simulink model "DC_MOTOR"  (R2016a)
settings: Solver=VariableStepAuto  StartTime=0.0  StopTime=tend  RelTol=1e-3
values from neighbouring files (symbols this model uses):
  c_M = 1.0    (= 1)    [DCTEST.m]    (also in a71test.m)
  J_A = 2.0    (= 2)    [DCTEST.m]    (also in a71test.m)
  L_A = 0.15    [DCTEST.m]    (also in a71test.m)
  Phi = 1.5    [DCTEST.m]    (also in a71test.m)
  R_A = 2.0    (= 2)    [DCTEST.m]    (also in a71test.m)
  t_ML_step = 12    [DCTEST.m]    (also in a71test.m = 3)
  t_u_A_step = 2    [DCTEST.m]
  u_A = 20    [DCTEST.m]    (also in a71test.m)
settings Model: Creator=mam1205  LastModifiedBy=mam1205

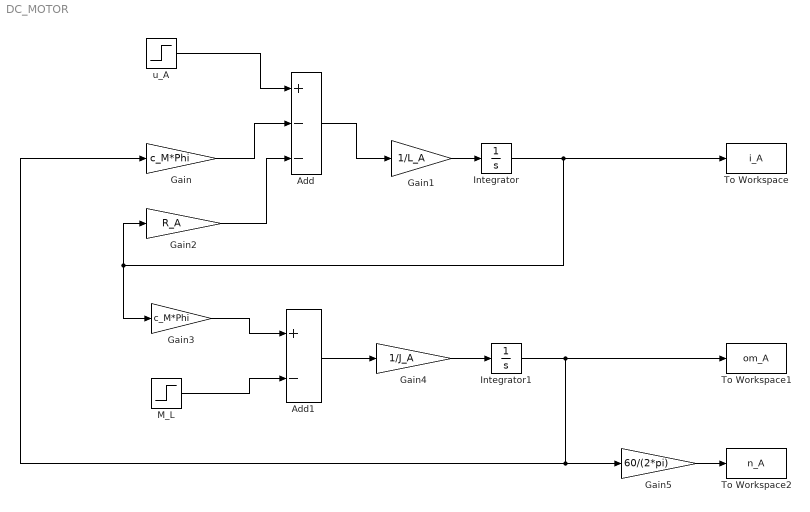
== system DC_MOTOR ==
  Add : Sum  Inputs=+--
  Add1 : Sum  Inputs=+-
  Gain : Gain  Gain=c_M*Phi
  Gain1 : Gain  Gain=1/L_A
  Gain2 : Gain  Gain=R_A
  Gain3 : Gain  Gain=c_M*Phi
  Gain4 : Gain  Gain=1/J_A
  Gain5 : Gain  Gain=60/(2*pi)
  Integrator : Integrator
  Integrator1 : Integrator
  "M_L " : Step  Time=t_ML_step  SampleTime=0
  To Workspace : ToWorkspace  VariableName=i_A  SaveFormat=Timeseries  SampleTime=-1
  To Workspace1 : ToWorkspace  VariableName=om_A  SaveFormat=Timeseries  SampleTime=-1
  To Workspace2 : ToWorkspace  VariableName=n_A  SaveFormat=Timeseries  SampleTime=-1
  u_A : Step  Time=t_u_A_step  After=u_A  SampleTime=0
  wires:
  Gain/1 -> Add/2
  u_A/1 -> Add/1
  Add/1 -> Gain1/1
  Gain1/1 -> Integrator/1
  Integrator/1 -> To Workspace/1, Gain2/1, Gain3/1
  Gain2/1 -> Add/3
  Gain3/1 -> Add1/1
  "M_L "/1 -> Add1/2
  Add1/1 -> Gain4/1
  Gain4/1 -> Integrator1/1
  Integrator1/1 -> Gain/1, Gain5/1, To Workspace1/1
  Gain5/1 -> To Workspace2/1
